simulink model "x2"  (R2016a)
settings: Solver=VariableStepAuto  StartTime=0.0  StopTime=50.0  RelTol=1e-3
settings Model: Creator=Arko  LastModifiedBy=Arko

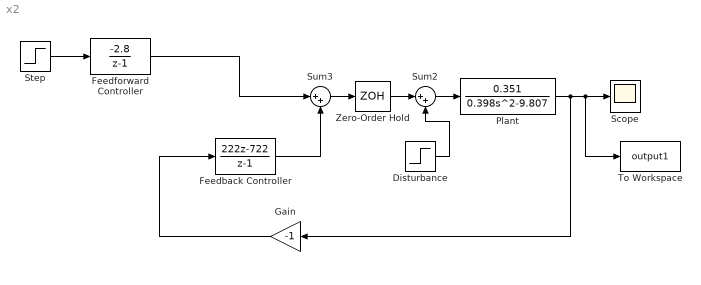
== system x2 ==
  Disturbance : Step  Time=0  After=0.1  SampleTime=0
  Feedback Controller : DiscreteTransferFcn  Numerator=[222 -722]  Denominator=[1 -1]  SampleTime=0.1
  Feedforward Controller : DiscreteTransferFcn  Numerator=[-2.8 ]  Denominator=[1 -1]  SampleTime=0.1
  Gain : Gain  Gain=-1
  Plant : TransferFcn  Numerator=[0 0.351]  Denominator="[0.398  0 -9.807]"
  Scope : Scope
  Step : Step  Time=0  SampleTime=0
  Sum2 : Sum  Inputs=|++
  Sum3 : Sum  Inputs=|++
  To Workspace : ToWorkspace  VariableName=output1  SampleTime=-1
  Zero-Order Hold : ZeroOrderHold  SampleTime=0.1
  wires:
  Plant/1 -> Gain/1, Scope/1, To Workspace/1
  Step/1 -> Feedforward Controller/1
  Sum3/1 -> Zero-Order Hold/1
  Feedback Controller/1 -> Sum3/2
  Feedforward Controller/1 -> Sum3/1
  Zero-Order Hold/1 -> Sum2/1
  Sum2/1 -> Plant/1
  Disturbance/1 -> Sum2/2
  Gain/1 -> Feedback Controller/1
